simulink model "logic111"  (R2020b)
settings: Solver=VariableStepAuto  StartTime=0.0  StopTime=10.0  RelTol=1e-3
libraries: simulink x5
settings Model: Creator=viett  LastModifiedBy=ASUS
settings DataIOCC: ReturnWorkspaceOutputs=off
settings DebuggingCC: ArithmeticOperatorsInVariantConditions=warning
settings SFSimCC: SimUseLocalCustomCode=off  CustomCodeUndefinedFunction=UseInterfaceOnly
settings RTWCC: RTWUseLocalCustomCode=off
settings CodeAppCC: StateflowObjectComments=on

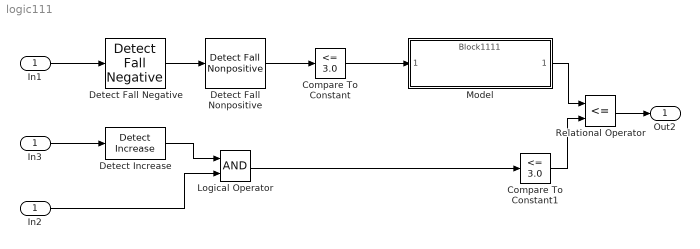
== system logic111 ==
  In1 : Inport
  Compare To Constant : simulink/Logic and Bit Operations/Compare To Constant  relop=<=  const=3.0  OutDataTypeStr=boolean
  Compare To Constant1 : simulink/Logic and Bit Operations/Compare To Constant  relop=<=  const=3.0  OutDataTypeStr=boolean
  Detect Increase : simulink/Logic and Bit Operations/Detect Increase  vinit=0.0  OutDataTypeStr=boolean
  Detect Fall Negative : simulink/Logic and Bit Operations/Detect Fall Negative  vinit=0  OutDataTypeStr=boolean
      settings: SourceProductBaseCode=SL
  Detect Fall Nonpositive : simulink/Logic and Bit Operations/Detect Fall Nonpositive  vinit=0  OutDataTypeStr=boolean
      settings: SourceProductBaseCode=SL
  In2 : InportShadow
  In3 : InportShadow
  Logical Operator : Logic  AllPortsSameDT=off  OutDataTypeStr=boolean
  Model : ModelReference  ModelNameDialog=Block1111.slx  SimulationMode=Normal  ModelReferenceVersion=1.4
  Relational Operator : RelationalOperator  Operator=<=  OutDataTypeStr=boolean  RndMeth=Simplest
  Out2 : Outport
  wires:
  Detect Fall Negative/1 -> Detect Fall Nonpositive/1
  Detect Fall Nonpositive/1 -> Compare To Constant/1
  Compare To Constant/1 -> Model/1
  In1/1 -> Detect Fall Negative/1
  Model/1 -> Relational Operator/1
  Logical Operator/1 -> Compare To Constant1/1
  In2/1 -> Logical Operator/2
  Compare To Constant1/1 -> Relational Operator/2
  Detect Increase/1 -> Logical Operator/1
  In3/1 -> Detect Increase/1
  Relational Operator/1 -> Out2/1
